simulink model "sm_DDPG_Training_Circuit_h1"  (R2022b)
settings: Solver=VariableStepAuto  StartTime=0.0  StopTime=2000  RelTol=1e-3
values from neighbouring files (symbols this model uses):
  areaFinEvap = 0.05    [pramInit.m]
  areaRoofRoom1 = roofArea/4    [pramInit.m]
  areaRoofRoom2 = roofArea/4    [pramInit.m]
  areaRoofRoom3 = roofArea/4    [pramInit.m]
  areaRoofRoom4 = roofArea/4    [pramInit.m]
  areaWallRoom1 = (lenHouse*3/5 *htHouse+widHouse*2/3*htHouse) - areaWindowRoom1    (= 95.6666666667)    [pramInit.m]
  areaWallRoom2 = (lenHouse*3/5*htHouse+widHouse/3*htHouse) - areaWindowRoom2    (= 83.3333333333)    [pramInit.m]
  areaWallRoom3 = (lenHouse*2/5*htHouse+widHouse*2/3*htHouse) - areaWindowRoom3    (= 72.6666666667)    [pramInit.m]
  areaWallRoom4 = (lenHouse*2/5*htHouse+widHouse/3*htHouse) - areaWindowRoom4    (= 59.3333333333)    [pramInit.m]
  areaWindowRoom1 = 3 * 1 *1    (= 3)    [pramInit.m]
  areaWindowRoom2 = 2 * 1 *1    (= 2)    [pramInit.m]
  areaWindowRoom3 = 2* 1 *1    (= 2)    [pramInit.m]
  areaWindowRoom4 = 2 * 1 *1    (= 2)    [pramInit.m]
  diaCond = 0.014    [pramInit.m]
  diaEvap = 0.126    [pramInit.m]
  diaGroundLoop = 0.032    [pramInit.m]
  diaOuterCond = 0.0158    [pramInit.m]
  diaOuterEvap = 0.1344    [pramInit.m]
  diaRadiatorPipe = 0.0125    [pramInit.m]
  htCondDuct = 0.3    [pramInit.m]
  htEvapDuct = 2.5    [pramInit.m]
  kTube = 400    [pramInit.m]
  leakRoofPercent = 0.1    [pramInit.m]
  leakWallPercent = 0.15    [pramInit.m]
  leakWinPercent = 0.2    [pramInit.m]
  numFinsEvap = 90    [pramInit.m]
  numTubeRowsCond = 20    [pramInit.m]
  numTubeRowsEvap = 400    [pramInit.m]
  numTubesPerRowCond = 10    [pramInit.m]
  numTubesPerRowEvap = 20    [pramInit.m]
  qGroundLoopPump = 18    [pramInit.m]
  roofDensity = 32    [pramInit.m]
  thkRoof = 0.2    [pramInit.m]
  thkWall = 0.2    [pramInit.m]
  thkWindow = 0.01    [pramInit.m]
  tInitHW = 50    [pramInit.m]
  tRoom = 23    [pramInit.m]
  Ts = hyper_agent_sample_time    [code_DDPG_Training.m]    (also in code_Experimental_Setup.m = 1)
  wallDensity = 1920    [pramInit.m]
  wCondDuct = 1.6    [pramInit.m]
  wEvapDuct = 0.96    [pramInit.m]
  windowDensity = 2700    [pramInit.m]
undefined symbols (not defined in the file or in its folder): DiscIntNeverNeededParam
libraries: fl_lib x144, nesl_utility x27, SimscapeFluids_lib x15, simulink x3, rllib x1
(part 3 of 4)

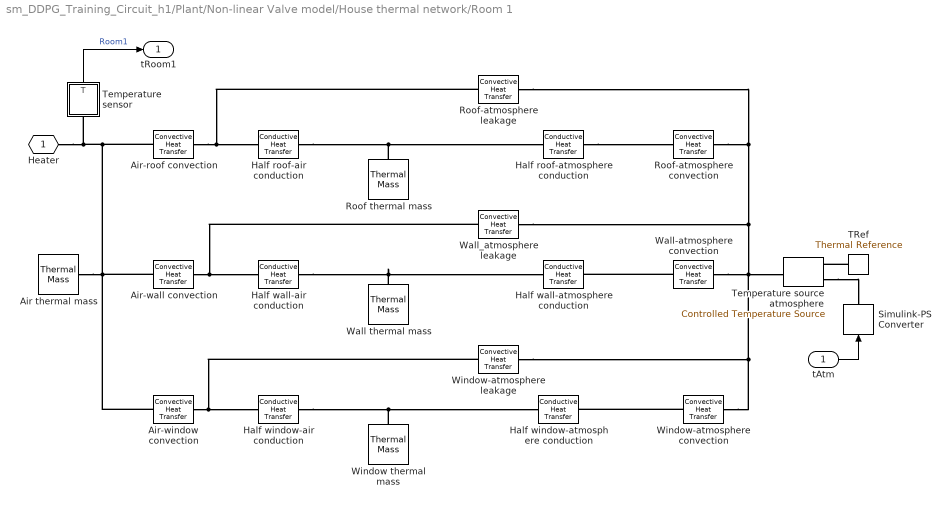
== system sm_DDPG_Training_Circuit_h1/Plant/Non-linear Valve model/House thermal network/Room 1 ==
  tAtm : Inport
  Air thermal mass : fl_lib/Thermal/Thermal Elements/Thermal Mass  mass=50 kg  sp_heat=cAir J/(K*kg)  num_ports=foundation.enum.numPorts2.one  T_specify=on  T_priority=Low  T=tRoom degC  T_nominal_specify=off  T_nominal_unit=K  T_nominal_value=1  Q_specify=off  Q_priority=High  Q=0 J/s  Q_nominal_specify=off  Q_nominal_unit=W  Q_nominal_value=1
  Air-roof convection : fl_lib/Thermal/Thermal Elements/Convective Heat Transfer  thermal_type=foundation.enum.constant_variable.constant  area=areaRoofRoom1 m^2  heat_tr_coeff=hAirRoof W/(m^2*K)  min_heat_tr_coeff=1e-3 W/(K*m^2)  T_specify=off  T_priority=None  T=0 K  T_nominal_specify=off  T_nominal_unit=K  T_nominal_value=1  Q_specify=off  Q_priority=None  Q=0 J/s  Q_nominal_specify=off  Q_nominal_unit=W  Q_nominal_value=1
  Air-wall convection : fl_lib/Thermal/Thermal Elements/Convective Heat Transfer  thermal_type=foundation.enum.constant_variable.constant  area=areaWallRoom1 m^2  heat_tr_coeff=hAirWall W/(m^2*K)  min_heat_tr_coeff=1e-3 W/(K*m^2)  T_specify=off  T_priority=None  T=0 K  T_nominal_specify=off  T_nominal_unit=K  T_nominal_value=1  Q_specify=off  Q_priority=None  Q=0 J/s  Q_nominal_specify=off  Q_nominal_unit=W  Q_nominal_value=1
  Air-window convection : fl_lib/Thermal/Thermal Elements/Convective Heat Transfer  thermal_type=foundation.enum.constant_variable.constant  area=areaWindowRoom1 m^2  heat_tr_coeff=hAirWindow W/(m^2*K)  min_heat_tr_coeff=1e-3 W/(K*m^2)  T_specify=off  T_priority=None  T=0 K  T_nominal_specify=off  T_nominal_unit=K  T_nominal_value=1  Q_specify=off  Q_priority=None  Q=0 J/s  Q_nominal_specify=off  Q_nominal_unit=W  Q_nominal_value=1
  Half roof-air conduction : fl_lib/Thermal/Thermal Elements/Conductive Heat Transfer  thermal_type=foundation.enum.ConstantVariableTabulated.Constant  wall_geometry=foundation.enum.ConductionWallGeometry.Planar  area=areaRoofRoom1 m^2  thickness=thkRoof/2 m  d_in=0.05 m  d_out=0.1 m  L=1 m  th_cond_min=10 W/(K*m)  th_cond=kRoof W/(m*K)  th_cond_TLU=[413, 401, 392, 383, 371, 357, 342] W/(K*m)  temp_TLU=[200, 273, 400, 600, 800, 1000, 1200] K  T_specify=off  T_priority=None  T=0 K  T_nominal_specify=off  T_nominal_unit=K  T_nominal_value=1  Q_specify=off  Q_priority=None  Q=0 J/s  Q_nominal_specify=off  Q_nominal_unit=W  Q_nominal_value=1
  Half roof-atmosphere conduction : fl_lib/Thermal/Thermal Elements/Conductive Heat Transfer  thermal_type=foundation.enum.ConstantVariableTabulated.Constant  wall_geometry=foundation.enum.ConductionWallGeometry.Planar  area=areaRoofRoom1 m^2  thickness=thkRoof/2 m  d_in=0.05 m  d_out=0.1 m  L=1 m  th_cond_min=10 W/(K*m)  th_cond=kRoof W/(m*K)  th_cond_TLU=[413, 401, 392, 383, 371, 357, 342] W/(K*m)  temp_TLU=[200, 273, 400, 600, 800, 1000, 1200] K  T_specify=off  T_priority=None  T=0 K  T_nominal_specify=off  T_nominal_unit=K  T_nominal_value=1  Q_specify=off  Q_priority=None  Q=0 J/s  Q_nominal_specify=off  Q_nominal_unit=W  Q_nominal_value=1
  Half wall-air conduction : fl_lib/Thermal/Thermal Elements/Conductive Heat Transfer  thermal_type=foundation.enum.ConstantVariableTabulated.Constant  wall_geometry=foundation.enum.ConductionWallGeometry.Planar  area=areaWallRoom1 m^2  thickness=thkWall/2 m  d_in=0.05 m  d_out=0.1 m  L=1 m  th_cond_min=10 W/(K*m)  th_cond=kWall W/(m*K)  th_cond_TLU=[413, 401, 392, 383, 371, 357, 342] W/(K*m)  temp_TLU=[200, 273, 400, 600, 800, 1000, 1200] K  T_specify=off  T_priority=None  T=0 K  T_nominal_specify=off  T_nominal_unit=K  T_nominal_value=1  Q_specify=off  Q_priority=None  Q=0 J/s  Q_nominal_specify=off  Q_nominal_unit=W  Q_nominal_value=1
  Half wall-atmosphere conduction : fl_lib/Thermal/Thermal Elements/Conductive Heat Transfer  thermal_type=foundation.enum.ConstantVariableTabulated.Constant  wall_geometry=foundation.enum.ConductionWallGeometry.Planar  area=areaWallRoom1 m^2  thickness=thkWall/2 m  d_in=0.05 m  d_out=0.1 m  L=1 m  th_cond_min=10 W/(K*m)  th_cond=kWall W/(m*K)  th_cond_TLU=[413, 401, 392, 383, 371, 357, 342] W/(K*m)  temp_TLU=[200, 273, 400, 600, 800, 1000, 1200] K  T_specify=off  T_priority=None  T=0 K  T_nominal_specify=off  T_nominal_unit=K  T_nominal_value=1  Q_specify=off  Q_priority=None  Q=0 J/s  Q_nominal_specify=off  Q_nominal_unit=W  Q_nominal_value=1
  Half window-air conduction : fl_lib/Thermal/Thermal Elements/Conductive Heat Transfer  thermal_type=foundation.enum.ConstantVariableTabulated.Constant  wall_geometry=foundation.enum.ConductionWallGeometry.Planar  area=areaWindowRoom1 m^2  thickness=thkWindow/2 m  d_in=0.05 m  d_out=0.1 m  L=1 m  th_cond_min=10 W/(K*m)  th_cond=kWindow W/(m*K)  th_cond_TLU=[413, 401, 392, 383, 371, 357, 342] W/(K*m)  temp_TLU=[200, 273, 400, 600, 800, 1000, 1200] K  T_specify=off  T_priority=None  T=0 K  T_nominal_specify=off  T_nominal_unit=K  T_nominal_value=1  Q_specify=off  Q_priority=None  Q=0 J/s  Q_nominal_specify=off  Q_nominal_unit=W  Q_nominal_value=1
  Half window-atmosphere conduction : fl_lib/Thermal/Thermal Elements/Conductive Heat Transfer  thermal_type=foundation.enum.ConstantVariableTabulated.Constant  wall_geometry=foundation.enum.ConductionWallGeometry.Planar  area=areaWindowRoom1 m^2  thickness=thkWindow/2 m  d_in=0.05 m  d_out=0.1 m  L=1 m  th_cond_min=10 W/(K*m)  th_cond=kWindow W/(m*K)  th_cond_TLU=[413, 401, 392, 383, 371, 357, 342] W/(K*m)  temp_TLU=[200, 273, 400, 600, 800, 1000, 1200] K  T_specify=off  T_priority=None  T=0 K  T_nominal_specify=off  T_nominal_unit=K  T_nominal_value=1  Q_specify=off  Q_priority=None  Q=0 J/s  Q_nominal_specify=off  Q_nominal_unit=W  Q_nominal_value=1
  Roof thermal mass : fl_lib/Thermal/Thermal Elements/Thermal Mass  mass=areaRoofRoom1*thkRoof*roofDensity kg  sp_heat=cRoof J/(K*kg)  num_ports=foundation.enum.numPorts2.one  T_specify=on  T_priority=Low  T=tRoom degC  T_nominal_specify=off  T_nominal_unit=K  T_nominal_value=1  Q_specify=off  Q_priority=None  Q=0 J/s  Q_nominal_specify=off  Q_nominal_unit=W  Q_nominal_value=1
  Roof-atmosphere convection : fl_lib/Thermal/Thermal Elements/Convective Heat Transfer  thermal_type=foundation.enum.constant_variable.constant  area=areaRoofRoom1 m^2  heat_tr_coeff=hRoofAtm W/(m^2*K)  min_heat_tr_coeff=1e-3 W/(K*m^2)  T_specify=off  T_priority=None  T=0 K  T_nominal_specify=off  T_nominal_unit=K  T_nominal_value=1  Q_specify=off  Q_priority=None  Q=0 J/s  Q_nominal_specify=off  Q_nominal_unit=W  Q_nominal_value=1
  Roof-atmosphere leakage : fl_lib/Thermal/Thermal Elements/Convective Heat Transfer  thermal_type=foundation.enum.constant_variable.constant  area=areaRoofRoom1*leakRoofPercent m^2  heat_tr_coeff=hRoofAtm W/(m^2*K)  min_heat_tr_coeff=1e-3 W/(K*m^2)  T_specify=off  T_priority=None  T=0 K  T_nominal_specify=off  T_nominal_unit=K  T_nominal_value=1  Q_specify=off  Q_priority=None  Q=0 J/s  Q_nominal_specify=off  Q_nominal_unit=W  Q_nominal_value=1
  Simulink-PS Converter : nesl_utility/Simulink-PS Converter  PhysicalDomain=network_engine_domain  SubClassName=ps_input  LeftPortType=input  RightPortType=output  PseudoPeriodic=off  Frequencies=[]  NoiseDistribution=none  NoiseParameters=[]  Unit=degC  AffineConversion=on  FilteringAndDerivatives=zero  SimscapeFilterOrder=1  InputFilterTimeConstant=.001  UdotUserProvided=1
  TRef : fl_lib/Thermal/Thermal Elements/Thermal Reference
  Temperature source atmosphere : fl_lib/Thermal/Thermal Sources/Controlled Temperature Source
  Temperature sensor : Subsystem
  Wall thermal mass : fl_lib/Thermal/Thermal Elements/Thermal Mass  mass=areaWallRoom1 * thkWall * wallDensity kg  sp_heat=cWall J/(K*kg)  num_ports=foundation.enum.numPorts2.one  T_specify=on  T_priority=Low  T=tRoom degC  T_nominal_specify=off  T_nominal_unit=K  T_nominal_value=1  Q_specify=off  Q_priority=Low  Q=0 J/s  Q_nominal_specify=off  Q_nominal_unit=W  Q_nominal_value=1
  Wall-atmosphere convection : fl_lib/Thermal/Thermal Elements/Convective Heat Transfer  thermal_type=foundation.enum.constant_variable.constant  area=areaWallRoom1 m^2  heat_tr_coeff=hWallAtm W/(m^2*K)  min_heat_tr_coeff=1e-3 W/(K*m^2)  T_specify=off  T_priority=None  T=0 K  T_nominal_specify=off  T_nominal_unit=K  T_nominal_value=1  Q_specify=off  Q_priority=None  Q=0 J/s  Q_nominal_specify=off  Q_nominal_unit=W  Q_nominal_value=1
  Wall_atmosphere leakage : fl_lib/Thermal/Thermal Elements/Convective Heat Transfer  thermal_type=foundation.enum.constant_variable.constant  area=areaWallRoom1*leakWallPercent m^2  heat_tr_coeff=hWallAtm W/(m^2*K)  min_heat_tr_coeff=1e-3 W/(K*m^2)  T_specify=off  T_priority=None  T=0 K  T_nominal_specify=off  T_nominal_unit=K  T_nominal_value=1  Q_specify=off  Q_priority=None  Q=0 J/s  Q_nominal_specify=off  Q_nominal_unit=W  Q_nominal_value=1
  Window thermal mass : fl_lib/Thermal/Thermal Elements/Thermal Mass  mass=areaWindowRoom1 * thkWindow * windowDensity kg  sp_heat=cWindow J/(K*kg)  num_ports=foundation.enum.numPorts2.one  T_specify=on  T_priority=Low  T=tRoom degC  T_nominal_specify=off  T_nominal_unit=K  T_nominal_value=1  Q_specify=off  Q_priority=None  Q=0 J/s  Q_nominal_specify=off  Q_nominal_unit=W  Q_nominal_value=1
  Window-atmosphere convection : fl_lib/Thermal/Thermal Elements/Convective Heat Transfer  thermal_type=foundation.enum.constant_variable.constant  area=areaWindowRoom1 m^2  heat_tr_coeff=hWindowAtm W/(m^2*K)  min_heat_tr_coeff=1e-3 W/(K*m^2)  T_specify=off  T_priority=None  T=0 K  T_nominal_specify=off  T_nominal_unit=K  T_nominal_value=1  Q_specify=off  Q_priority=None  Q=0 J/s  Q_nominal_specify=off  Q_nominal_unit=W  Q_nominal_value=1
  Window-atmosphere leakage : fl_lib/Thermal/Thermal Elements/Convective Heat Transfer  thermal_type=foundation.enum.constant_variable.constant  area=areaWindowRoom1*leakWinPercent m^2  heat_tr_coeff=hWindowAtm W/(m^2*K)  min_heat_tr_coeff=1e-3 W/(K*m^2)  T_specify=off  T_priority=None  T=0 K  T_nominal_specify=off  T_nominal_unit=K  T_nominal_value=1  Q_specify=off  Q_priority=None  Q=0 J/s  Q_nominal_specify=off  Q_nominal_unit=W  Q_nominal_value=1
  Heater : PMIOPort  Tag=PMCPort  Side=Left
  tRoom1 : Outport  VectorParamsAs1DForOutWhenUnconnected=off
  wires:
  Temperature sensor/1(T) -> tRoom1/1  "Room1"
  tAtm/1 -> Simulink-PS Converter/1
  connections:
  Temperature sensor/LConn1 -- Air-window convection/LConn1 -- Air thermal mass/LConn1 -- Air-wall convection/LConn1 -- Air-roof convection/LConn1 -- Heater/RConn1
  TRef/LConn1 -- Temperature source atmosphere/RConn2
  Half wall-air conduction/RConn1 -- Half wall-atmosphere conduction/LConn1 -- Wall thermal mass/LConn1
  Half window-air conduction/RConn1 -- Window thermal mass/LConn1 -- Half window-atmosphere conduction/LConn1
  Half roof-air conduction/RConn1 -- Half roof-atmosphere conduction/LConn1 -- Roof thermal mass/LConn1
  Air-wall convection/RConn1 -- Wall_atmosphere leakage/LConn1 -- Half wall-air conduction/LConn1
  Air-window convection/RConn1 -- Window-atmosphere leakage/LConn1 -- Half window-air conduction/LConn1
  Wall-atmosphere convection/LConn1 -- Half wall-atmosphere conduction/RConn1
  Window-atmosphere convection/LConn1 -- Half window-atmosphere conduction/RConn1
  Air-roof convection/RConn1 -- Roof-atmosphere leakage/LConn1 -- Half roof-air conduction/LConn1
  Temperature source atmosphere/RConn1 -- Simulink-PS Converter/RConn1
  Half roof-atmosphere conduction/RConn1 -- Roof-atmosphere convection/LConn1
  Wall-atmosphere convection/RConn1 -- Window-atmosphere leakage/RConn1 -- Window-atmosphere convection/RConn1 -- Wall_atmosphere leakage/RConn1 -- Roof-atmosphere convection/RConn1 -- Roof-atmosphere leakage/RConn1 -- Temperature source atmosphere/LConn1

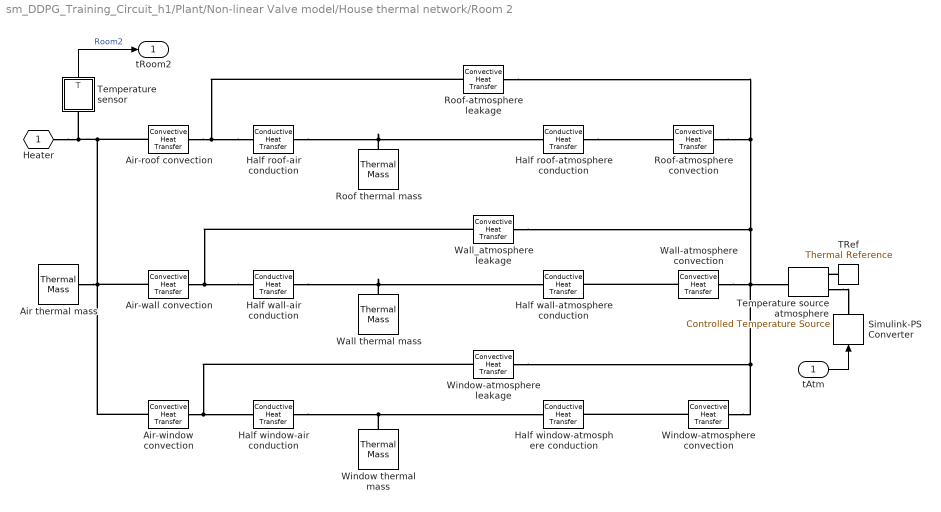
== system sm_DDPG_Training_Circuit_h1/Plant/Non-linear Valve model/House thermal network/Room 2 ==
  tAtm : Inport
  Air thermal mass : fl_lib/Thermal/Thermal Elements/Thermal Mass  mass=50 kg  sp_heat=cAir J/(K*kg)  num_ports=foundation.enum.numPorts2.one  T_specify=on  T_priority=Low  T=tRoom degC  T_nominal_specify=off  T_nominal_unit=K  T_nominal_value=1  Q_specify=off  Q_priority=High  Q=0 J/s  Q_nominal_specify=off  Q_nominal_unit=W  Q_nominal_value=1
  Air-roof convection : fl_lib/Thermal/Thermal Elements/Convective Heat Transfer  thermal_type=foundation.enum.constant_variable.constant  area=areaRoofRoom2 m^2  heat_tr_coeff=hAirRoof W/(m^2*K)  min_heat_tr_coeff=1e-3 W/(K*m^2)  T_specify=off  T_priority=None  T=0 K  T_nominal_specify=off  T_nominal_unit=K  T_nominal_value=1  Q_specify=off  Q_priority=None  Q=0 J/s  Q_nominal_specify=off  Q_nominal_unit=W  Q_nominal_value=1
  Air-wall convection : fl_lib/Thermal/Thermal Elements/Convective Heat Transfer  thermal_type=foundation.enum.constant_variable.constant  area=areaWallRoom2 m^2  heat_tr_coeff=hAirWall W/(m^2*K)  min_heat_tr_coeff=1e-3 W/(K*m^2)  T_specify=off  T_priority=None  T=0 K  T_nominal_specify=off  T_nominal_unit=K  T_nominal_value=1  Q_specify=off  Q_priority=None  Q=0 J/s  Q_nominal_specify=off  Q_nominal_unit=W  Q_nominal_value=1
  Air-window convection : fl_lib/Thermal/Thermal Elements/Convective Heat Transfer  thermal_type=foundation.enum.constant_variable.constant  area=areaWindowRoom2 m^2  heat_tr_coeff=hAirWindow W/(m^2*K)  min_heat_tr_coeff=1e-3 W/(K*m^2)  T_specify=off  T_priority=None  T=0 K  T_nominal_specify=off  T_nominal_unit=K  T_nominal_value=1  Q_specify=off  Q_priority=None  Q=0 J/s  Q_nominal_specify=off  Q_nominal_unit=W  Q_nominal_value=1
  Half roof-air conduction : fl_lib/Thermal/Thermal Elements/Conductive Heat Transfer  thermal_type=foundation.enum.ConstantVariableTabulated.Constant  wall_geometry=foundation.enum.ConductionWallGeometry.Planar  area=areaRoofRoom2 m^2  thickness=thkRoof/2 m  d_in=0.05 m  d_out=0.1 m  L=1 m  th_cond_min=10 W/(K*m)  th_cond=kRoof W/(m*K)  th_cond_TLU=[413, 401, 392, 383, 371, 357, 342] W/(K*m)  temp_TLU=[200, 273, 400, 600, 800, 1000, 1200] K  T_specify=off  T_priority=None  T=0 K  T_nominal_specify=off  T_nominal_unit=K  T_nominal_value=1  Q_specify=off  Q_priority=None  Q=0 J/s  Q_nominal_specify=off  Q_nominal_unit=W  Q_nominal_value=1
  Half roof-atmosphere conduction : fl_lib/Thermal/Thermal Elements/Conductive Heat Transfer  thermal_type=foundation.enum.ConstantVariableTabulated.Constant  wall_geometry=foundation.enum.ConductionWallGeometry.Planar  area=areaRoofRoom2 m^2  thickness=thkRoof/2 m  d_in=0.05 m  d_out=0.1 m  L=1 m  th_cond_min=10 W/(K*m)  th_cond=kRoof W/(m*K)  th_cond_TLU=[413, 401, 392, 383, 371, 357, 342] W/(K*m)  temp_TLU=[200, 273, 400, 600, 800, 1000, 1200] K  T_specify=off  T_priority=None  T=0 K  T_nominal_specify=off  T_nominal_unit=K  T_nominal_value=1  Q_specify=off  Q_priority=None  Q=0 J/s  Q_nominal_specify=off  Q_nominal_unit=W  Q_nominal_value=1
  Half wall-air conduction : fl_lib/Thermal/Thermal Elements/Conductive Heat Transfer  thermal_type=foundation.enum.ConstantVariableTabulated.Constant  wall_geometry=foundation.enum.ConductionWallGeometry.Planar  area=areaWallRoom2 m^2  thickness=thkWall/2 m  d_in=0.05 m  d_out=0.1 m  L=1 m  th_cond_min=10 W/(K*m)  th_cond=kWall W/(m*K)  th_cond_TLU=[413, 401, 392, 383, 371, 357, 342] W/(K*m)  temp_TLU=[200, 273, 400, 600, 800, 1000, 1200] K  T_specify=off  T_priority=None  T=0 K  T_nominal_specify=off  T_nominal_unit=K  T_nominal_value=1  Q_specify=off  Q_priority=None  Q=0 J/s  Q_nominal_specify=off  Q_nominal_unit=W  Q_nominal_value=1
  Half wall-atmosphere conduction : fl_lib/Thermal/Thermal Elements/Conductive Heat Transfer  thermal_type=foundation.enum.ConstantVariableTabulated.Constant  wall_geometry=foundation.enum.ConductionWallGeometry.Planar  area=areaWallRoom2 m^2  thickness=thkWall/2 m  d_in=0.05 m  d_out=0.1 m  L=1 m  th_cond_min=10 W/(K*m)  th_cond=kWall W/(m*K)  th_cond_TLU=[413, 401, 392, 383, 371, 357, 342] W/(K*m)  temp_TLU=[200, 273, 400, 600, 800, 1000, 1200] K  T_specify=off  T_priority=None  T=0 K  T_nominal_specify=off  T_nominal_unit=K  T_nominal_value=1  Q_specify=off  Q_priority=None  Q=0 J/s  Q_nominal_specify=off  Q_nominal_unit=W  Q_nominal_value=1
  Half window-air conduction : fl_lib/Thermal/Thermal Elements/Conductive Heat Transfer  thermal_type=foundation.enum.ConstantVariableTabulated.Constant  wall_geometry=foundation.enum.ConductionWallGeometry.Planar  area=areaWindowRoom2 m^2  thickness=thkWindow/2 m  d_in=0.05 m  d_out=0.1 m  L=1 m  th_cond_min=10 W/(K*m)  th_cond=kWindow W/(m*K)  th_cond_TLU=[413, 401, 392, 383, 371, 357, 342] W/(K*m)  temp_TLU=[200, 273, 400, 600, 800, 1000, 1200] K  T_specify=off  T_priority=None  T=0 K  T_nominal_specify=off  T_nominal_unit=K  T_nominal_value=1  Q_specify=off  Q_priority=None  Q=0 J/s  Q_nominal_specify=off  Q_nominal_unit=W  Q_nominal_value=1
  Half window-atmosphere conduction : fl_lib/Thermal/Thermal Elements/Conductive Heat Transfer  thermal_type=foundation.enum.ConstantVariableTabulated.Constant  wall_geometry=foundation.enum.ConductionWallGeometry.Planar  area=areaWindowRoom2 m^2  thickness=thkWindow/2 m  d_in=0.05 m  d_out=0.1 m  L=1 m  th_cond_min=10 W/(K*m)  th_cond=kWindow W/(m*K)  th_cond_TLU=[413, 401, 392, 383, 371, 357, 342] W/(K*m)  temp_TLU=[200, 273, 400, 600, 800, 1000, 1200] K  T_specify=off  T_priority=None  T=0 K  T_nominal_specify=off  T_nominal_unit=K  T_nominal_value=1  Q_specify=off  Q_priority=None  Q=0 J/s  Q_nominal_specify=off  Q_nominal_unit=W  Q_nominal_value=1
  Roof thermal mass : fl_lib/Thermal/Thermal Elements/Thermal Mass  mass=areaRoofRoom2*thkRoof*roofDensity kg  sp_heat=cRoof J/(K*kg)  num_ports=foundation.enum.numPorts2.one  T_specify=on  T_priority=Low  T=tRoom degC  T_nominal_specify=off  T_nominal_unit=K  T_nominal_value=1  Q_specify=off  Q_priority=None  Q=0 J/s  Q_nominal_specify=off  Q_nominal_unit=W  Q_nominal_value=1
  Roof-atmosphere convection : fl_lib/Thermal/Thermal Elements/Convective Heat Transfer  thermal_type=foundation.enum.constant_variable.constant  area=areaRoofRoom2 m^2  heat_tr_coeff=hRoofAtm W/(m^2*K)  min_heat_tr_coeff=1e-3 W/(K*m^2)  T_specify=off  T_priority=None  T=0 K  T_nominal_specify=off  T_nominal_unit=K  T_nominal_value=1  Q_specify=off  Q_priority=None  Q=0 J/s  Q_nominal_specify=off  Q_nominal_unit=W  Q_nominal_value=1
  Roof-atmosphere leakage : fl_lib/Thermal/Thermal Elements/Convective Heat Transfer  thermal_type=foundation.enum.constant_variable.constant  area=areaRoofRoom2*leakRoofPercent m^2  heat_tr_coeff=hRoofAtm W/(m^2*K)  min_heat_tr_coeff=1e-3 W/(K*m^2)  T_specify=off  T_priority=None  T=0 K  T_nominal_specify=off  T_nominal_unit=K  T_nominal_value=1  Q_specify=off  Q_priority=None  Q=0 J/s  Q_nominal_specify=off  Q_nominal_unit=W  Q_nominal_value=1
  Simulink-PS Converter : nesl_utility/Simulink-PS Converter  PhysicalDomain=network_engine_domain  SubClassName=ps_input  LeftPortType=input  RightPortType=output  PseudoPeriodic=off  Frequencies=[]  NoiseDistribution=none  NoiseParameters=[]  Unit=degC  AffineConversion=on  FilteringAndDerivatives=zero  SimscapeFilterOrder=1  InputFilterTimeConstant=.001  UdotUserProvided=1
  TRef : fl_lib/Thermal/Thermal Elements/Thermal Reference
  Temperature source atmosphere : fl_lib/Thermal/Thermal Sources/Controlled Temperature Source
  Temperature sensor : Subsystem
  Wall thermal mass : fl_lib/Thermal/Thermal Elements/Thermal Mass  mass=areaWallRoom2 * thkWall * wallDensity kg  sp_heat=cWall J/(K*kg)  num_ports=foundation.enum.numPorts2.one  T_specify=on  T_priority=Low  T=tRoom degC  T_nominal_specify=off  T_nominal_unit=K  T_nominal_value=1  Q_specify=off  Q_priority=None  Q=0 J/s  Q_nominal_specify=off  Q_nominal_unit=W  Q_nominal_value=1
  Wall-atmosphere convection : fl_lib/Thermal/Thermal Elements/Convective Heat Transfer  thermal_type=foundation.enum.constant_variable.constant  area=areaWallRoom2 m^2  heat_tr_coeff=hWallAtm W/(m^2*K)  min_heat_tr_coeff=1e-3 W/(K*m^2)  T_specify=off  T_priority=None  T=0 K  T_nominal_specify=off  T_nominal_unit=K  T_nominal_value=1  Q_specify=off  Q_priority=None  Q=0 J/s  Q_nominal_specify=off  Q_nominal_unit=W  Q_nominal_value=1
  Wall_atmosphere leakage : fl_lib/Thermal/Thermal Elements/Convective Heat Transfer  thermal_type=foundation.enum.constant_variable.constant  area=areaWallRoom2*leakWallPercent m^2  heat_tr_coeff=hWallAtm W/(m^2*K)  min_heat_tr_coeff=1e-3 W/(K*m^2)  T_specify=off  T_priority=None  T=0 K  T_nominal_specify=off  T_nominal_unit=K  T_nominal_value=1  Q_specify=off  Q_priority=None  Q=0 J/s  Q_nominal_specify=off  Q_nominal_unit=W  Q_nominal_value=1
  Window thermal mass : fl_lib/Thermal/Thermal Elements/Thermal Mass  mass=areaWindowRoom2 * thkWindow * windowDensity kg  sp_heat=cWindow J/(K*kg)  num_ports=foundation.enum.numPorts2.one  T_specify=on  T_priority=Low  T=tRoom degC  T_nominal_specify=off  T_nominal_unit=K  T_nominal_value=1  Q_specify=off  Q_priority=None  Q=0 J/s  Q_nominal_specify=off  Q_nominal_unit=W  Q_nominal_value=1
  Window-atmosphere convection : fl_lib/Thermal/Thermal Elements/Convective Heat Transfer  thermal_type=foundation.enum.constant_variable.constant  area=areaWindowRoom2 m^2  heat_tr_coeff=hWindowAtm W/(m^2*K)  min_heat_tr_coeff=1e-3 W/(K*m^2)  T_specify=off  T_priority=None  T=0 K  T_nominal_specify=off  T_nominal_unit=K  T_nominal_value=1  Q_specify=off  Q_priority=None  Q=0 J/s  Q_nominal_specify=off  Q_nominal_unit=W  Q_nominal_value=1
  Window-atmosphere leakage : fl_lib/Thermal/Thermal Elements/Convective Heat Transfer  thermal_type=foundation.enum.constant_variable.constant  area=areaWindowRoom2*leakWinPercent m^2  heat_tr_coeff=hWindowAtm W/(m^2*K)  min_heat_tr_coeff=1e-3 W/(K*m^2)  T_specify=off  T_priority=None  T=0 K  T_nominal_specify=off  T_nominal_unit=K  T_nominal_value=1  Q_specify=off  Q_priority=None  Q=0 J/s  Q_nominal_specify=off  Q_nominal_unit=W  Q_nominal_value=1
  Heater : PMIOPort  Tag=PMCPort  Side=Left
  tRoom2 : Outport  VectorParamsAs1DForOutWhenUnconnected=off
  wires:
  Temperature sensor/1(T) -> tRoom2/1  "Room2"
  tAtm/1 -> Simulink-PS Converter/1
  connections:
  Air-roof convection/LConn1 -- Air thermal mass/LConn1 -- Air-wall convection/LConn1 -- Air-window convection/LConn1 -- Heater/RConn1 -- Temperature sensor/LConn1
  Wall thermal mass/LConn1 -- Half wall-atmosphere conduction/LConn1 -- Half wall-air conduction/RConn1
  Window thermal mass/LConn1 -- Half window-atmosphere conduction/LConn1 -- Half window-air conduction/RConn1
  Roof thermal mass/LConn1 -- Half roof-atmosphere conduction/LConn1 -- Half roof-air conduction/RConn1
  Wall-atmosphere convection/RConn1 -- Window-atmosphere leakage/RConn1 -- Window-atmosphere convection/RConn1 -- Roof-atmosphere leakage/RConn1 -- Roof-atmosphere convection/RConn1 -- Wall_atmosphere leakage/RConn1 -- Temperature source atmosphere/LConn1
  Half wall-air conduction/LConn1 -- Air-wall convection/RConn1 -- Wall_atmosphere leakage/LConn1
  Air-window convection/RConn1 -- Window-atmosphere leakage/LConn1 -- Half window-air conduction/LConn1
  Half roof-air conduction/LConn1 -- Air-roof convection/RConn1 -- Roof-atmosphere leakage/LConn1
  Wall-atmosphere convection/LConn1 -- Half wall-atmosphere conduction/RConn1
  Window-atmosphere convection/LConn1 -- Half window-atmosphere conduction/RConn1
  Half roof-atmosphere conduction/RConn1 -- Roof-atmosphere convection/LConn1
  TRef/LConn1 -- Temperature source atmosphere/RConn2
  Temperature source atmosphere/RConn1 -- Simulink-PS Converter/RConn1

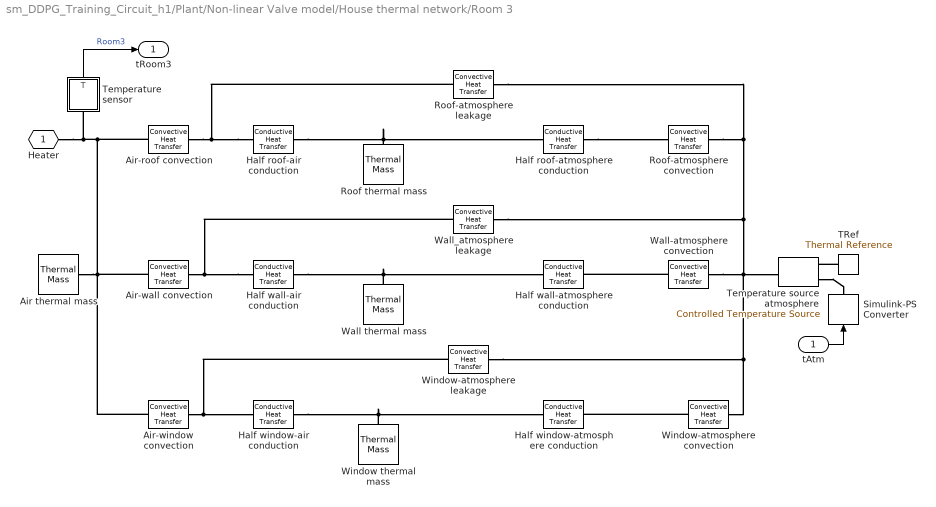
== system sm_DDPG_Training_Circuit_h1/Plant/Non-linear Valve model/House thermal network/Room 3 ==
  tAtm : Inport
  Air thermal mass : fl_lib/Thermal/Thermal Elements/Thermal Mass  mass=50 kg  sp_heat=cAir J/(K*kg)  num_ports=foundation.enum.numPorts2.one  T_specify=on  T_priority=Low  T=tRoom degC  T_nominal_specify=off  T_nominal_unit=K  T_nominal_value=1  Q_specify=off  Q_priority=High  Q=0 J/s  Q_nominal_specify=off  Q_nominal_unit=W  Q_nominal_value=1
  Air-roof convection : fl_lib/Thermal/Thermal Elements/Convective Heat Transfer  thermal_type=foundation.enum.constant_variable.constant  area=areaRoofRoom3 m^2  heat_tr_coeff=hAirRoof W/(m^2*K)  min_heat_tr_coeff=1e-3 W/(K*m^2)  T_specify=off  T_priority=None  T=0 K  T_nominal_specify=off  T_nominal_unit=K  T_nominal_value=1  Q_specify=off  Q_priority=None  Q=0 J/s  Q_nominal_specify=off  Q_nominal_unit=W  Q_nominal_value=1
  Air-wall convection : fl_lib/Thermal/Thermal Elements/Convective Heat Transfer  thermal_type=foundation.enum.constant_variable.constant  area=areaWallRoom3 m^2  heat_tr_coeff=hAirWall W/(m^2*K)  min_heat_tr_coeff=1e-3 W/(K*m^2)  T_specify=off  T_priority=None  T=0 K  T_nominal_specify=off  T_nominal_unit=K  T_nominal_value=1  Q_specify=off  Q_priority=None  Q=0 J/s  Q_nominal_specify=off  Q_nominal_unit=W  Q_nominal_value=1
  Air-window convection : fl_lib/Thermal/Thermal Elements/Convective Heat Transfer  thermal_type=foundation.enum.constant_variable.constant  area=areaWindowRoom3 m^2  heat_tr_coeff=hAirWindow W/(m^2*K)  min_heat_tr_coeff=1e-3 W/(K*m^2)  T_specify=off  T_priority=None  T=0 K  T_nominal_specify=off  T_nominal_unit=K  T_nominal_value=1  Q_specify=off  Q_priority=None  Q=0 J/s  Q_nominal_specify=off  Q_nominal_unit=W  Q_nominal_value=1
  Half roof-air conduction : fl_lib/Thermal/Thermal Elements/Conductive Heat Transfer  thermal_type=foundation.enum.ConstantVariableTabulated.Constant  wall_geometry=foundation.enum.ConductionWallGeometry.Planar  area=areaRoofRoom3 m^2  thickness=thkRoof/2 m  d_in=0.05 m  d_out=0.1 m  L=1 m  th_cond_min=10 W/(K*m)  th_cond=kRoof W/(m*K)  th_cond_TLU=[413, 401, 392, 383, 371, 357, 342] W/(K*m)  temp_TLU=[200, 273, 400, 600, 800, 1000, 1200] K  T_specify=off  T_priority=None  T=0 K  T_nominal_specify=off  T_nominal_unit=K  T_nominal_value=1  Q_specify=off  Q_priority=None  Q=0 J/s  Q_nominal_specify=off  Q_nominal_unit=W  Q_nominal_value=1
  Half roof-atmosphere conduction : fl_lib/Thermal/Thermal Elements/Conductive Heat Transfer  thermal_type=foundation.enum.ConstantVariableTabulated.Constant  wall_geometry=foundation.enum.ConductionWallGeometry.Planar  area=areaRoofRoom3 m^2  thickness=thkRoof/2 m  d_in=0.05 m  d_out=0.1 m  L=1 m  th_cond_min=10 W/(K*m)  th_cond=kRoof W/(m*K)  th_cond_TLU=[413, 401, 392, 383, 371, 357, 342] W/(K*m)  temp_TLU=[200, 273, 400, 600, 800, 1000, 1200] K  T_specify=off  T_priority=None  T=0 K  T_nominal_specify=off  T_nominal_unit=K  T_nominal_value=1  Q_specify=off  Q_priority=None  Q=0 J/s  Q_nominal_specify=off  Q_nominal_unit=W  Q_nominal_value=1
  Half wall-air conduction : fl_lib/Thermal/Thermal Elements/Conductive Heat Transfer  thermal_type=foundation.enum.ConstantVariableTabulated.Constant  wall_geometry=foundation.enum.ConductionWallGeometry.Planar  area=areaWallRoom3 m^2  thickness=thkWall/2 m  d_in=0.05 m  d_out=0.1 m  L=1 m  th_cond_min=10 W/(K*m)  th_cond=kWall W/(m*K)  th_cond_TLU=[413, 401, 392, 383, 371, 357, 342] W/(K*m)  temp_TLU=[200, 273, 400, 600, 800, 1000, 1200] K  T_specify=off  T_priority=None  T=0 K  T_nominal_specify=off  T_nominal_unit=K  T_nominal_value=1  Q_specify=off  Q_priority=None  Q=0 J/s  Q_nominal_specify=off  Q_nominal_unit=W  Q_nominal_value=1
  Half wall-atmosphere conduction : fl_lib/Thermal/Thermal Elements/Conductive Heat Transfer  thermal_type=foundation.enum.ConstantVariableTabulated.Constant  wall_geometry=foundation.enum.ConductionWallGeometry.Planar  area=areaWallRoom3 m^2  thickness=thkWall/2 m  d_in=0.05 m  d_out=0.1 m  L=1 m  th_cond_min=10 W/(K*m)  th_cond=kWall W/(m*K)  th_cond_TLU=[413, 401, 392, 383, 371, 357, 342] W/(K*m)  temp_TLU=[200, 273, 400, 600, 800, 1000, 1200] K  T_specify=off  T_priority=None  T=0 K  T_nominal_specify=off  T_nominal_unit=K  T_nominal_value=1  Q_specify=off  Q_priority=None  Q=0 J/s  Q_nominal_specify=off  Q_nominal_unit=W  Q_nominal_value=1
  Half window-air conduction : fl_lib/Thermal/Thermal Elements/Conductive Heat Transfer  thermal_type=foundation.enum.ConstantVariableTabulated.Constant  wall_geometry=foundation.enum.ConductionWallGeometry.Planar  area=areaWindowRoom3 m^2  thickness=thkWindow/2 m  d_in=0.05 m  d_out=0.1 m  L=1 m  th_cond_min=10 W/(K*m)  th_cond=kWindow W/(m*K)  th_cond_TLU=[413, 401, 392, 383, 371, 357, 342] W/(K*m)  temp_TLU=[200, 273, 400, 600, 800, 1000, 1200] K  T_specify=off  T_priority=None  T=0 K  T_nominal_specify=off  T_nominal_unit=K  T_nominal_value=1  Q_specify=off  Q_priority=None  Q=0 J/s  Q_nominal_specify=off  Q_nominal_unit=W  Q_nominal_value=1
  Half window-atmosphere conduction : fl_lib/Thermal/Thermal Elements/Conductive Heat Transfer  thermal_type=foundation.enum.ConstantVariableTabulated.Constant  wall_geometry=foundation.enum.ConductionWallGeometry.Planar  area=areaWindowRoom3 m^2  thickness=thkWindow/2 m  d_in=0.05 m  d_out=0.1 m  L=1 m  th_cond_min=10 W/(K*m)  th_cond=kWindow W/(m*K)  th_cond_TLU=[413, 401, 392, 383, 371, 357, 342] W/(K*m)  temp_TLU=[200, 273, 400, 600, 800, 1000, 1200] K  T_specify=off  T_priority=None  T=0 K  T_nominal_specify=off  T_nominal_unit=K  T_nominal_value=1  Q_specify=off  Q_priority=None  Q=0 J/s  Q_nominal_specify=off  Q_nominal_unit=W  Q_nominal_value=1
  Roof thermal mass : fl_lib/Thermal/Thermal Elements/Thermal Mass  mass=areaRoofRoom3*thkRoof*roofDensity kg  sp_heat=cRoof J/(K*kg)  num_ports=foundation.enum.numPorts2.one  T_specify=on  T_priority=Low  T=tRoom degC  T_nominal_specify=off  T_nominal_unit=K  T_nominal_value=1  Q_specify=off  Q_priority=None  Q=0 J/s  Q_nominal_specify=off  Q_nominal_unit=W  Q_nominal_value=1
  Roof-atmosphere convection : fl_lib/Thermal/Thermal Elements/Convective Heat Transfer  thermal_type=foundation.enum.constant_variable.constant  area=areaRoofRoom3 m^2  heat_tr_coeff=hRoofAtm W/(m^2*K)  min_heat_tr_coeff=1e-3 W/(K*m^2)  T_specify=off  T_priority=None  T=0 K  T_nominal_specify=off  T_nominal_unit=K  T_nominal_value=1  Q_specify=off  Q_priority=None  Q=0 J/s  Q_nominal_specify=off  Q_nominal_unit=W  Q_nominal_value=1
  Roof-atmosphere leakage : fl_lib/Thermal/Thermal Elements/Convective Heat Transfer  thermal_type=foundation.enum.constant_variable.constant  area=areaRoofRoom3*leakRoofPercent m^2  heat_tr_coeff=hRoofAtm W/(m^2*K)  min_heat_tr_coeff=1e-3 W/(K*m^2)  T_specify=off  T_priority=None  T=0 K  T_nominal_specify=off  T_nominal_unit=K  T_nominal_value=1  Q_specify=off  Q_priority=None  Q=0 J/s  Q_nominal_specify=off  Q_nominal_unit=W  Q_nominal_value=1
  Simulink-PS Converter : nesl_utility/Simulink-PS Converter  PhysicalDomain=network_engine_domain  SubClassName=ps_input  LeftPortType=input  RightPortType=output  PseudoPeriodic=off  Frequencies=[]  NoiseDistribution=none  NoiseParameters=[]  Unit=degC  AffineConversion=on  FilteringAndDerivatives=zero  SimscapeFilterOrder=1  InputFilterTimeConstant=.001  UdotUserProvided=1
  TRef : fl_lib/Thermal/Thermal Elements/Thermal Reference
  Temperature source atmosphere : fl_lib/Thermal/Thermal Sources/Controlled Temperature Source
  Temperature sensor : Subsystem
  Wall thermal mass : fl_lib/Thermal/Thermal Elements/Thermal Mass  mass=areaWallRoom3 * thkWall * wallDensity kg  sp_heat=cWall J/(K*kg)  num_ports=foundation.enum.numPorts2.one  T_specify=on  T_priority=Low  T=tRoom degC  T_nominal_specify=off  T_nominal_unit=K  T_nominal_value=1  Q_specify=off  Q_priority=None  Q=0 J/s  Q_nominal_specify=off  Q_nominal_unit=W  Q_nominal_value=1
  Wall-atmosphere convection : fl_lib/Thermal/Thermal Elements/Convective Heat Transfer  thermal_type=foundation.enum.constant_variable.constant  area=areaWallRoom3 m^2  heat_tr_coeff=hWallAtm W/(m^2*K)  min_heat_tr_coeff=1e-3 W/(K*m^2)  T_specify=off  T_priority=None  T=0 K  T_nominal_specify=off  T_nominal_unit=K  T_nominal_value=1  Q_specify=off  Q_priority=None  Q=0 J/s  Q_nominal_specify=off  Q_nominal_unit=W  Q_nominal_value=1
  Wall_atmosphere leakage : fl_lib/Thermal/Thermal Elements/Convective Heat Transfer  thermal_type=foundation.enum.constant_variable.constant  area=areaWallRoom3*leakWallPercent m^2  heat_tr_coeff=hWallAtm W/(m^2*K)  min_heat_tr_coeff=1e-3 W/(K*m^2)  T_specify=off  T_priority=None  T=0 K  T_nominal_specify=off  T_nominal_unit=K  T_nominal_value=1  Q_specify=off  Q_priority=None  Q=0 J/s  Q_nominal_specify=off  Q_nominal_unit=W  Q_nominal_value=1
  Window thermal mass : fl_lib/Thermal/Thermal Elements/Thermal Mass  mass=areaWindowRoom3 * thkWindow * windowDensity kg  sp_heat=cWindow J/(K*kg)  num_ports=foundation.enum.numPorts2.one  T_specify=on  T_priority=Low  T=tRoom degC  T_nominal_specify=off  T_nominal_unit=K  T_nominal_value=1  Q_specify=off  Q_priority=None  Q=0 J/s  Q_nominal_specify=off  Q_nominal_unit=W  Q_nominal_value=1
  Window-atmosphere convection : fl_lib/Thermal/Thermal Elements/Convective Heat Transfer  thermal_type=foundation.enum.constant_variable.constant  area=areaWindowRoom3 m^2  heat_tr_coeff=hWindowAtm W/(m^2*K)  min_heat_tr_coeff=1e-3 W/(K*m^2)  T_specify=off  T_priority=None  T=0 K  T_nominal_specify=off  T_nominal_unit=K  T_nominal_value=1  Q_specify=off  Q_priority=None  Q=0 J/s  Q_nominal_specify=off  Q_nominal_unit=W  Q_nominal_value=1
  Window-atmosphere leakage : fl_lib/Thermal/Thermal Elements/Convective Heat Transfer  thermal_type=foundation.enum.constant_variable.constant  area=areaWindowRoom3*leakWinPercent m^2  heat_tr_coeff=hWindowAtm W/(m^2*K)  min_heat_tr_coeff=1e-3 W/(K*m^2)  T_specify=off  T_priority=None  T=0 K  T_nominal_specify=off  T_nominal_unit=K  T_nominal_value=1  Q_specify=off  Q_priority=None  Q=0 J/s  Q_nominal_specify=off  Q_nominal_unit=W  Q_nominal_value=1
  Heater : PMIOPort  Tag=PMCPort  Side=Left
  tRoom3 : Outport  VectorParamsAs1DForOutWhenUnconnected=off
  wires:
  Temperature sensor/1(T) -> tRoom3/1  "Room3"
  tAtm/1 -> Simulink-PS Converter/1
  connections:
  Air-roof convection/LConn1 -- Air thermal mass/LConn1 -- Air-wall convection/LConn1 -- Air-window convection/LConn1 -- Heater/RConn1 -- Temperature sensor/LConn1
  Wall thermal mass/LConn1 -- Half wall-atmosphere conduction/LConn1 -- Half wall-air conduction/RConn1
  Window thermal mass/LConn1 -- Half window-atmosphere conduction/LConn1 -- Half window-air conduction/RConn1
  Half roof-air conduction/RConn1 -- Half roof-atmosphere conduction/LConn1 -- Roof thermal mass/LConn1
  Half wall-air conduction/LConn1 -- Air-wall convection/RConn1 -- Wall_atmosphere leakage/LConn1
  Air-window convection/RConn1 -- Window-atmosphere leakage/LConn1 -- Half window-air conduction/LConn1
  Half roof-air conduction/LConn1 -- Air-roof convection/RConn1 -- Roof-atmosphere leakage/LConn1
  TRef/LConn1 -- Temperature source atmosphere/RConn2
  Wall-atmosphere convection/LConn1 -- Half wall-atmosphere conduction/RConn1
  Half roof-atmosphere conduction/RConn1 -- Roof-atmosphere convection/LConn1
  Window-atmosphere convection/LConn1 -- Half window-atmosphere conduction/RConn1
  Temperature source atmosphere/RConn1 -- Simulink-PS Converter/RConn1
  Wall-atmosphere convection/RConn1 -- Window-atmosphere leakage/RConn1 -- Window-atmosphere convection/RConn1 -- Roof-atmosphere convection/RConn1 -- Roof-atmosphere leakage/RConn1 -- Wall_atmosphere leakage/RConn1 -- Temperature source atmosphere/LConn1

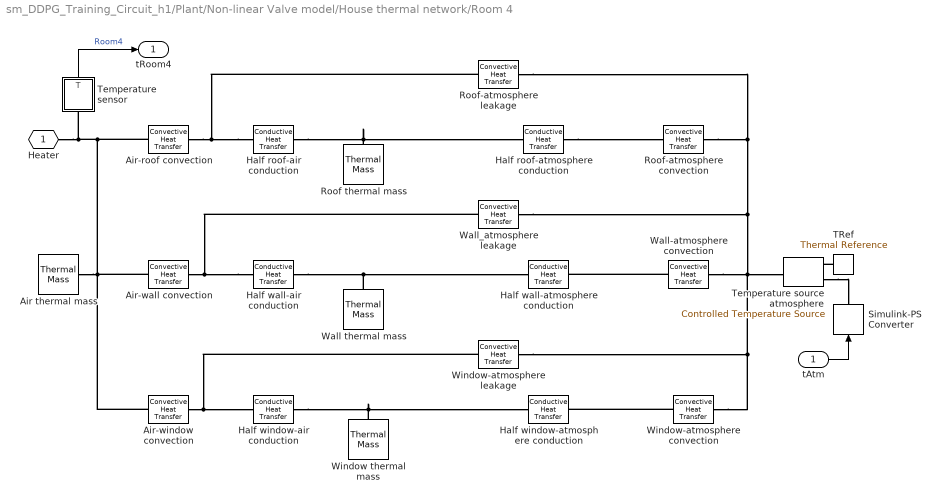
== system sm_DDPG_Training_Circuit_h1/Plant/Non-linear Valve model/House thermal network/Room 4 ==
  tAtm : Inport
  Air thermal mass : fl_lib/Thermal/Thermal Elements/Thermal Mass  mass=50 kg  sp_heat=cAir J/(K*kg)  num_ports=foundation.enum.numPorts2.one  T_specify=on  T_priority=Low  T=tRoom degC  T_nominal_specify=off  T_nominal_unit=K  T_nominal_value=1  Q_specify=off  Q_priority=High  Q=0 J/s  Q_nominal_specify=off  Q_nominal_unit=W  Q_nominal_value=1
  Air-roof convection : fl_lib/Thermal/Thermal Elements/Convective Heat Transfer  thermal_type=foundation.enum.constant_variable.constant  area=areaRoofRoom4 m^2  heat_tr_coeff=hAirRoof W/(m^2*K)  min_heat_tr_coeff=1e-3 W/(K*m^2)  T_specify=off  T_priority=None  T=0 K  T_nominal_specify=off  T_nominal_unit=K  T_nominal_value=1  Q_specify=off  Q_priority=None  Q=0 J/s  Q_nominal_specify=off  Q_nominal_unit=W  Q_nominal_value=1
  Air-wall convection : fl_lib/Thermal/Thermal Elements/Convective Heat Transfer  thermal_type=foundation.enum.constant_variable.constant  area=areaWallRoom4 m^2  heat_tr_coeff=hAirWall W/(m^2*K)  min_heat_tr_coeff=1e-3 W/(K*m^2)  T_specify=off  T_priority=None  T=0 K  T_nominal_specify=off  T_nominal_unit=K  T_nominal_value=1  Q_specify=off  Q_priority=None  Q=0 J/s  Q_nominal_specify=off  Q_nominal_unit=W  Q_nominal_value=1
  Air-window convection : fl_lib/Thermal/Thermal Elements/Convective Heat Transfer  thermal_type=foundation.enum.constant_variable.constant  area=areaWindowRoom4 m^2  heat_tr_coeff=hAirWindow W/(m^2*K)  min_heat_tr_coeff=1e-3 W/(K*m^2)  T_specify=off  T_priority=None  T=0 K  T_nominal_specify=off  T_nominal_unit=K  T_nominal_value=1  Q_specify=off  Q_priority=None  Q=0 J/s  Q_nominal_specify=off  Q_nominal_unit=W  Q_nominal_value=1
  Half roof-air conduction : fl_lib/Thermal/Thermal Elements/Conductive Heat Transfer  thermal_type=foundation.enum.ConstantVariableTabulated.Constant  wall_geometry=foundation.enum.ConductionWallGeometry.Planar  area=areaRoofRoom4 m^2  thickness=thkRoof/2 m  d_in=0.05 m  d_out=0.1 m  L=1 m  th_cond_min=10 W/(K*m)  th_cond=kRoof W/(m*K)  th_cond_TLU=[413, 401, 392, 383, 371, 357, 342] W/(K*m)  temp_TLU=[200, 273, 400, 600, 800, 1000, 1200] K  T_specify=off  T_priority=None  T=0 K  T_nominal_specify=off  T_nominal_unit=K  T_nominal_value=1  Q_specify=off  Q_priority=None  Q=0 J/s  Q_nominal_specify=off  Q_nominal_unit=W  Q_nominal_value=1
  Half roof-atmosphere conduction : fl_lib/Thermal/Thermal Elements/Conductive Heat Transfer  thermal_type=foundation.enum.ConstantVariableTabulated.Constant  wall_geometry=foundation.enum.ConductionWallGeometry.Planar  area=areaRoofRoom4 m^2  thickness=thkRoof/2 m  d_in=0.05 m  d_out=0.1 m  L=1 m  th_cond_min=10 W/(K*m)  th_cond=kRoof W/(m*K)  th_cond_TLU=[413, 401, 392, 383, 371, 357, 342] W/(K*m)  temp_TLU=[200, 273, 400, 600, 800, 1000, 1200] K  T_specify=off  T_priority=None  T=0 K  T_nominal_specify=off  T_nominal_unit=K  T_nominal_value=1  Q_specify=off  Q_priority=None  Q=0 J/s  Q_nominal_specify=off  Q_nominal_unit=W  Q_nominal_value=1
  Half wall-air conduction : fl_lib/Thermal/Thermal Elements/Conductive Heat Transfer  thermal_type=foundation.enum.ConstantVariableTabulated.Constant  wall_geometry=foundation.enum.ConductionWallGeometry.Planar  area=areaWallRoom4 m^2  thickness=thkWall/2 m  d_in=0.05 m  d_out=0.1 m  L=1 m  th_cond_min=10 W/(K*m)  th_cond=kWall W/(m*K)  th_cond_TLU=[413, 401, 392, 383, 371, 357, 342] W/(K*m)  temp_TLU=[200, 273, 400, 600, 800, 1000, 1200] K  T_specify=off  T_priority=None  T=0 K  T_nominal_specify=off  T_nominal_unit=K  T_nominal_value=1  Q_specify=off  Q_priority=None  Q=0 J/s  Q_nominal_specify=off  Q_nominal_unit=W  Q_nominal_value=1
  Half wall-atmosphere conduction : fl_lib/Thermal/Thermal Elements/Conductive Heat Transfer  thermal_type=foundation.enum.ConstantVariableTabulated.Constant  wall_geometry=foundation.enum.ConductionWallGeometry.Planar  area=areaWallRoom4 m^2  thickness=thkWall/2 m  d_in=0.05 m  d_out=0.1 m  L=1 m  th_cond_min=10 W/(K*m)  th_cond=kWall W/(m*K)  th_cond_TLU=[413, 401, 392, 383, 371, 357, 342] W/(K*m)  temp_TLU=[200, 273, 400, 600, 800, 1000, 1200] K  T_specify=off  T_priority=None  T=0 K  T_nominal_specify=off  T_nominal_unit=K  T_nominal_value=1  Q_specify=off  Q_priority=None  Q=0 J/s  Q_nominal_specify=off  Q_nominal_unit=W  Q_nominal_value=1
  Half window-air conduction : fl_lib/Thermal/Thermal Elements/Conductive Heat Transfer  thermal_type=foundation.enum.ConstantVariableTabulated.Constant  wall_geometry=foundation.enum.ConductionWallGeometry.Planar  area=areaWindowRoom4 m^2  thickness=thkWindow/2 m  d_in=0.05 m  d_out=0.1 m  L=1 m  th_cond_min=10 W/(K*m)  th_cond=kWindow W/(m*K)  th_cond_TLU=[413, 401, 392, 383, 371, 357, 342] W/(K*m)  temp_TLU=[200, 273, 400, 600, 800, 1000, 1200] K  T_specify=off  T_priority=None  T=0 K  T_nominal_specify=off  T_nominal_unit=K  T_nominal_value=1  Q_specify=off  Q_priority=None  Q=0 J/s  Q_nominal_specify=off  Q_nominal_unit=W  Q_nominal_value=1
  Half window-atmosphere conduction : fl_lib/Thermal/Thermal Elements/Conductive Heat Transfer  thermal_type=foundation.enum.ConstantVariableTabulated.Constant  wall_geometry=foundation.enum.ConductionWallGeometry.Planar  area=areaWindowRoom4 m^2  thickness=thkWindow/2 m  d_in=0.05 m  d_out=0.1 m  L=1 m  th_cond_min=10 W/(K*m)  th_cond=kWindow W/(m*K)  th_cond_TLU=[413, 401, 392, 383, 371, 357, 342] W/(K*m)  temp_TLU=[200, 273, 400, 600, 800, 1000, 1200] K  T_specify=off  T_priority=None  T=0 K  T_nominal_specify=off  T_nominal_unit=K  T_nominal_value=1  Q_specify=off  Q_priority=None  Q=0 J/s  Q_nominal_specify=off  Q_nominal_unit=W  Q_nominal_value=1
  Roof thermal mass : fl_lib/Thermal/Thermal Elements/Thermal Mass  mass=areaRoofRoom4*thkRoof*roofDensity kg  sp_heat=cRoof J/(K*kg)  num_ports=foundation.enum.numPorts2.one  T_specify=on  T_priority=Low  T=tRoom degC  T_nominal_specify=off  T_nominal_unit=K  T_nominal_value=1  Q_specify=off  Q_priority=None  Q=0 J/s  Q_nominal_specify=off  Q_nominal_unit=W  Q_nominal_value=1
  Roof-atmosphere convection : fl_lib/Thermal/Thermal Elements/Convective Heat Transfer  thermal_type=foundation.enum.constant_variable.constant  area=areaRoofRoom4 m^2  heat_tr_coeff=hRoofAtm W/(m^2*K)  min_heat_tr_coeff=1e-3 W/(K*m^2)  T_specify=off  T_priority=None  T=0 K  T_nominal_specify=off  T_nominal_unit=K  T_nominal_value=1  Q_specify=off  Q_priority=None  Q=0 J/s  Q_nominal_specify=off  Q_nominal_unit=W  Q_nominal_value=1
  Roof-atmosphere leakage : fl_lib/Thermal/Thermal Elements/Convective Heat Transfer  thermal_type=foundation.enum.constant_variable.constant  area=areaRoofRoom4*leakRoofPercent m^2  heat_tr_coeff=hRoofAtm W/(m^2*K)  min_heat_tr_coeff=1e-3 W/(K*m^2)  T_specify=off  T_priority=None  T=0 K  T_nominal_specify=off  T_nominal_unit=K  T_nominal_value=1  Q_specify=off  Q_priority=None  Q=0 J/s  Q_nominal_specify=off  Q_nominal_unit=W  Q_nominal_value=1
  Simulink-PS Converter : nesl_utility/Simulink-PS Converter  PhysicalDomain=network_engine_domain  SubClassName=ps_input  LeftPortType=input  RightPortType=output  PseudoPeriodic=off  Frequencies=[]  NoiseDistribution=none  NoiseParameters=[]  Unit=degC  AffineConversion=on  FilteringAndDerivatives=zero  SimscapeFilterOrder=1  InputFilterTimeConstant=.001  UdotUserProvided=1
  TRef : fl_lib/Thermal/Thermal Elements/Thermal Reference
  Temperature source atmosphere : fl_lib/Thermal/Thermal Sources/Controlled Temperature Source
  Temperature sensor : Subsystem
  Wall thermal mass : fl_lib/Thermal/Thermal Elements/Thermal Mass  mass=areaWallRoom4 * thkWall * wallDensity kg  sp_heat=cWall J/(K*kg)  num_ports=foundation.enum.numPorts2.one  T_specify=on  T_priority=Low  T=tRoom degC  T_nominal_specify=off  T_nominal_unit=K  T_nominal_value=1  Q_specify=off  Q_priority=None  Q=0 J/s  Q_nominal_specify=off  Q_nominal_unit=W  Q_nominal_value=1
  Wall-atmosphere convection : fl_lib/Thermal/Thermal Elements/Convective Heat Transfer  thermal_type=foundation.enum.constant_variable.constant  area=areaWallRoom4 m^2  heat_tr_coeff=hWallAtm W/(m^2*K)  min_heat_tr_coeff=1e-3 W/(K*m^2)  T_specify=off  T_priority=None  T=0 K  T_nominal_specify=off  T_nominal_unit=K  T_nominal_value=1  Q_specify=off  Q_priority=None  Q=0 J/s  Q_nominal_specify=off  Q_nominal_unit=W  Q_nominal_value=1
  Wall_atmosphere leakage : fl_lib/Thermal/Thermal Elements/Convective Heat Transfer  thermal_type=foundation.enum.constant_variable.constant  area=areaWallRoom4*leakWallPercent m^2  heat_tr_coeff=hWallAtm W/(m^2*K)  min_heat_tr_coeff=1e-3 W/(K*m^2)  T_specify=off  T_priority=None  T=0 K  T_nominal_specify=off  T_nominal_unit=K  T_nominal_value=1  Q_specify=off  Q_priority=None  Q=0 J/s  Q_nominal_specify=off  Q_nominal_unit=W  Q_nominal_value=1
  Window thermal mass : fl_lib/Thermal/Thermal Elements/Thermal Mass  mass=areaWindowRoom4 * thkWindow * windowDensity kg  sp_heat=cWindow J/(K*kg)  num_ports=foundation.enum.numPorts2.one  T_specify=on  T_priority=Low  T=tRoom degC  T_nominal_specify=off  T_nominal_unit=K  T_nominal_value=1  Q_specify=off  Q_priority=None  Q=0 J/s  Q_nominal_specify=off  Q_nominal_unit=W  Q_nominal_value=1
  Window-atmosphere convection : fl_lib/Thermal/Thermal Elements/Convective Heat Transfer  thermal_type=foundation.enum.constant_variable.constant  area=areaWindowRoom4 m^2  heat_tr_coeff=hWindowAtm W/(m^2*K)  min_heat_tr_coeff=1e-3 W/(K*m^2)  T_specify=off  T_priority=None  T=0 K  T_nominal_specify=off  T_nominal_unit=K  T_nominal_value=1  Q_specify=off  Q_priority=None  Q=0 J/s  Q_nominal_specify=off  Q_nominal_unit=W  Q_nominal_value=1
  Window-atmosphere leakage : fl_lib/Thermal/Thermal Elements/Convective Heat Transfer  thermal_type=foundation.enum.constant_variable.constant  area=areaWindowRoom4*leakWinPercent m^2  heat_tr_coeff=hWindowAtm W/(m^2*K)  min_heat_tr_coeff=1e-3 W/(K*m^2)  T_specify=off  T_priority=None  T=0 K  T_nominal_specify=off  T_nominal_unit=K  T_nominal_value=1  Q_specify=off  Q_priority=None  Q=0 J/s  Q_nominal_specify=off  Q_nominal_unit=W  Q_nominal_value=1
  Heater : PMIOPort  Tag=PMCPort  Side=Left
  tRoom4 : Outport  VectorParamsAs1DForOutWhenUnconnected=off
  wires:
  Temperature sensor/1(T) -> tRoom4/1  "Room4"
  tAtm/1 -> Simulink-PS Converter/1
  connections:
  Temperature sensor/LConn1 -- Air-roof convection/LConn1 -- Air thermal mass/LConn1 -- Air-wall convection/LConn1 -- Air-window convection/LConn1 -- Heater/RConn1
  Half window-air conduction/RConn1 -- Half window-atmosphere conduction/LConn1 -- Window thermal mass/LConn1
  Half roof-air conduction/RConn1 -- Half roof-atmosphere conduction/LConn1 -- Roof thermal mass/LConn1
  Wall-atmosphere convection/RConn1 -- Window-atmosphere leakage/RConn1 -- Window-atmosphere convection/RConn1 -- Roof-atmosphere leakage/RConn1 -- Roof-atmosphere convection/RConn1 -- Wall_atmosphere leakage/RConn1 -- Temperature source atmosphere/LConn1
  Half wall-air conduction/LConn1 -- Air-wall convection/RConn1 -- Wall_atmosphere leakage/LConn1
  Air-window convection/RConn1 -- Window-atmosphere leakage/LConn1 -- Half window-air conduction/LConn1
  Half roof-air conduction/LConn1 -- Air-roof convection/RConn1 -- Roof-atmosphere leakage/LConn1
  TRef/LConn1 -- Temperature source atmosphere/RConn2
  Temperature source atmosphere/RConn1 -- Simulink-PS Converter/RConn1
  Window-atmosphere convection/LConn1 -- Half window-atmosphere conduction/RConn1
  Half roof-atmosphere conduction/RConn1 -- Roof-atmosphere convection/LConn1
  Wall-atmosphere convection/LConn1 -- Half wall-atmosphere conduction/RConn1
  Half wall-air conduction/RConn1 -- Wall thermal mass/LConn1 -- Half wall-atmosphere conduction/LConn1

== system sm_DDPG_Training_Circuit_h1/Plant/Non-linear Valve model/House thermal network/Room 1/Temperature sensor ==
  PS2S : nesl_utility/PS-Simulink Converter  PhysicalDomain=network_engine_domain  SubClassName=ps_output  LeftPortType=input  RightPortType=output  PseudoPeriodic=off  Frequencies=[]  VectorFormat=1-D array  Unit=degC  AffineConversion=on
  TRef : fl_lib/Thermal/Thermal Elements/Thermal Reference
  Temperature Sensor : fl_lib/Thermal/Thermal Sensors/Temperature Sensor
  Pr : PMIOPort  Side=Left
  T : Outport  VectorParamsAs1DForOutWhenUnconnected=off
  wires:
  PS2S/1 -> T/1
  connections:
  Pr/RConn1 -- Temperature Sensor/LConn1
  PS2S/LConn1 -- Temperature Sensor/RConn2
  Temperature Sensor/RConn1 -- TRef/LConn1
